simulink model "justtest"  (R2023a)
settings: Solver=ode5  StartTime=0.0  StopTime=inf  RelTol=1e-3
libraries: instrumentseriallib x3, svdutilitieslib x1, etargetslib x1
settings Model: Creator=arian  LastModifiedBy=arian
settings DebuggingCC: ParameterPrecisionLossMsg=none
settings HardwareCC: ProdBitPerLong=64  ProdHWDeviceType=Intel->x86-64 (Linux 64)
settings RTWCC: Description=Simulink Desktop Real-Time  SystemTargetFile=sldrt.tlc  TemplateMakefile=sldrt.tmf  RTWCompilerOptimization=on
settings CodeAppCC: MaxIdLength=95
settings SimulinkDesktopRealTimeCC: TargetLibSuffix=_sldrt.a  TargetPreCompLibLocation=C:\Program Files\MATLAB\R2023a\toolbox\sldrt\lib\win64

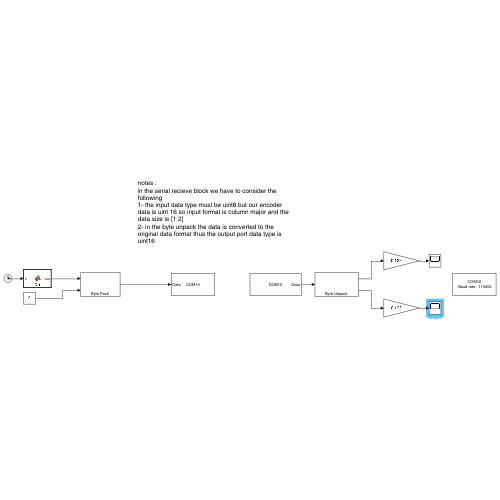
[thumbnail: Simulink's stored preview of the top-level diagram]
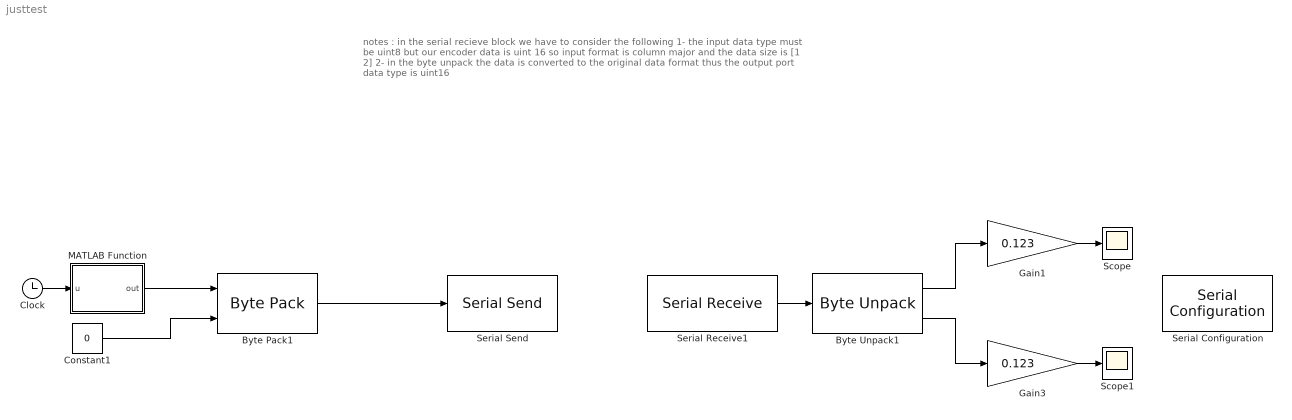
== system justtest ==
  note: notes :
      | in the serial recieve block we have to consider the following
      | 1- the input data type must be uint8 but our encoder data is uint 16 so input format is column major and the data size is [1 2]
      | 2- in the byte unpack the data is converted to the original data format thus the output port data type is uint16
  Byte Pack1 : svdutilitieslib/Byte Pack  maskPackedDataType=uint8  datatypes={'uint8';'uint8'}  byteAlign=1  blockPlatform=arduinoert
  Byte Unpack1 : etargetslib/Byte Unpack  dimensions={[1],[1]}  datatypes={'int16','int16'}  byteAlign=1
      settings: LibrarySourceBlock=embeddedtargetslib/Host Communication/Byte Unpack
  Clock : Clock
      settings: Decimation=300
  Constant1 : Constant  Value=0  OutDataTypeStr=uint8
  Gain1 : Gain  Gain=0.123  OutDataTypeStr=int32
  Gain3 : Gain  Gain=0.123  OutDataTypeStr=int32
  MATLAB Function : MATLAB Function  TreatAsAtomicUnit=on
  Scope : Scope
  Scope1 : Scope
  Serial Configuration : instrumentseriallib/Serial Configuration  Priority=-200000  PortSel=COM10  Port=COM10  ComPort=COM10  BaudRate=115200  DataBits=8  Parity=none  StopBits=1  ByteOrder=little-endian  FlowControl=none  Timeout=10  SimulateUsing=Interpreted execution  BlockInModel=on  aMode=1
      settings: LibrarySourceBlock=embeddedtargetslib/Host Communication/Serial Configuration
  Serial Receive1 : instrumentseriallib/Serial Receive  Priority=1  PortSel=COM10  Port=COM10  ComPort=COM10  DataType=uint8  SaveDataType=uint8  ToggleHeader=off  Header=[]  ToggleTerminator=off  Terminator=<none>  CustomTerminator=[]  InputFormat=Column major  ToggleDataSize=on  DataSize=[2 2]  EnableBlockingMode=on  ActionDataUnavailable=Output last received value  ActionWhenDataUnavailable=Output last received value  CustomValue=0  SampleTime=0.01  SimulateUsing=Interpreted execution  BlockInModel=on  aMode=1
  Serial Send : instrumentseriallib/Serial Send  Priority=1  PortSel=COM10  Port=COM10  ComPort=COM10  Header=[]  Terminator=<none>  CustomTerminator=[]  EnableBlockingMode=off  SimulateUsing=Interpreted execution  BlockInModel=on  aMode=1
      settings: LibrarySourceBlock=embeddedtargetslib/Host Communication/Serial Send
  wires:
  Serial Receive1/1 -> Byte Unpack1/1
  Constant1/1 -> Byte Pack1/2
  MATLAB Function/1(out) -> Byte Pack1/1
  Byte Unpack1/1 -> Gain1/1
  Byte Unpack1/2 -> Gain3/1
  Byte Pack1/1 -> Serial Send/1
  Clock/1 -> MATLAB Function/1(u)
  Gain3/1 -> Scope1/1
  Gain1/1 -> Scope/1

== matlab function justtest/MATLAB Function ==
  data: u input; out output
function out = fcn(u)
    if u < 5
        y = 50;
    elseif u < 7
        y = 0;
    elseif u < 10
        y = 45;
    elseif u < 12 
        y = 0;
    elseif u < 14
        y = 60;
    elseif u < 16
        y = 65;
    else
        y = 0;
    end
out =uint8(y) ;
